simulink model "eBooster_48v_Gen2_r2009a"  (Simulink 7.6)
settings: Solver=FixedStepDiscrete  StartTime=0.0  StopTime=0.2  FixedStep=T_sim  RelTol=1e-3
InitFcn:
  | init_simulation
values from neighbouring files (symbols this model uses):
  C_Load = 0    [init_MIL.m]    (also in init_simulation.m)
  curr_adc_gain = 0.6247    [init_MIL.m]    (also in init_simulation.m)
  en_avr = 0    [init_MIL.m]    (also in init_simulation.m)
  FOC_CURR_GAIN_SCU10 = 640    [init_MIL.m]    (also in init_simulation.m)
  FOC_CURR_NULLIFICATION = 511    [init_MIL.m]    (also in init_simulation.m)
  I_max = 106    [init_MIL.m]    (also in init_simulation.m = 100; plot_current_limits.m = 160)
  Id_ref_min = -1*160*0.8    (= -128)    [init_MIL.m]    (also in init_simulation.m)
  J_motor = (3.2220 + 11.438)*1e-6    (= 1.466e-05)    [init_MIL.m]    (also in init_simulation.m)
  Kpi = 0.3    [init_MIL.m]    (also in init_simulation.m)
  Kpi_n = 0.0015    [init_MIL.m]    (also in init_simulation.m)
  load_motor_spd_ramp = (load_motor_target_spd - load_motor_start_spd)/spd_ramp_time    (= 62831.8530718)    [init_MIL.m]    (also in init_simulation.m)
  load_motor_start_spd = 40000*2*pi/60    (= 4188.79020479)    [init_MIL.m]    (also in init_simulation.m)
  load_motor_target_spd = 70000*2*pi/60    (= 7330.38285838)    [init_MIL.m]    (also in init_simulation.m)
  Ls = 17.05e-6/3    (= 5.68333333333e-06)    [init_MIL.m]    (also in init_simulation.m; plot_current_limits.m)
  N_avr = 1    [init_MIL.m]    (also in init_simulation.m)
  Nset_const = 50000    [init_MIL.m]    (also in init_simulation.m)
  ONEDIVSQRT3_SCU16 = 37837    [init_MIL.m]    (also in init_simulation.m)
  Pp = 1    [init_MIL.m]    (also in init_simulation.m; plot_current_limits.m)
  psi_p = 5.3e-3/sqrt(3)*0.95    [init_MIL.m]    (also in init_simulation.m)
  Rs = 10e-3*(1+0.0039*(120-20))/3    (= 0.00463333333333)    [init_MIL.m]    (also in init_simulation.m; plot_current_limits.m)
  Sel_Bench_Mode = 1    [init_MIL.m]    (also in init_simulation.m)
  Sel_Bench_Spd = 0    [init_MIL.m]    (also in init_simulation.m)
  Sel_id_ref = 2    [init_MIL.m]    (also in init_simulation.m)
  Sel_Load = 1    [init_MIL.m]    (also in init_simulation.m)
  sel_udq = 0    [init_simulation.m]
  Set_Speed_rpm = 50000    [init_MIL.m]    (also in init_simulation.m)
  T_ctrl = T_pwm    (= 3.57002606119e-05)    [init_MIL.m]    (also in init_simulation.m)
  T_LUT_T = [0.1864, 0.1969, 0.2092, 0.2230, 0.2381, 0.2541, 0.2709, 0.2880, 0.3054, 0.3226, 0.3395, 0.3557, 0.3710, 0.3851, 0.3978, 0.4088, 0.4178 ... (first row only)    [init_MIL.m]    (also in init_simulation.m)
  T_sim = T_pwm/100    (= 3.57002606119e-07)    [init_MIL.m]    (also in init_simulation.m)
  Tni = Ts    (= 0.00122661870504)    [init_MIL.m]    (also in init_simulation.m)
  Tni_n = Ts*1.5    (= 0.00183992805755)    [init_MIL.m]    (also in init_simulation.m)
  V_dc = 36    [init_MIL.m]    (also in init_simulation.m)
libraries: simulink x27
(part 1 of 2)
Description:
  | This model can be used to document and simulate the eBooster_Gen2_48V application including:
  | - Control algorithm
  | - Fix point scaling
  | - Interfaces (function arguments, global variables...)
  | 
  | File history:
settings Model: Creator=tree5_000  LastModifiedBy=meng
settings CodeAppCC: CustomSymbolStrType=$N$R$M_T

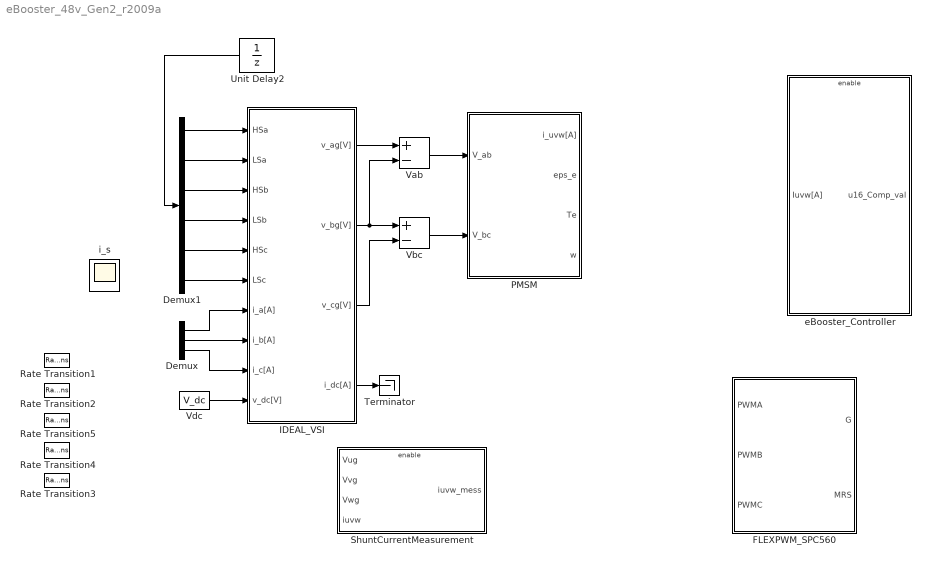
== system eBooster_48v_Gen2_r2009a ==
  Demux : Demux  Outputs=3
  Demux1 : Demux  Outputs=6
  FLEXPWM_SPC560 : Subsystem
  IDEAL_VSI : Subsystem
  PMSM : Subsystem  MinMaxOverflowLogging=ForceOff
  Rate Transition{1..5} (5 alike) : RateTransition  Integrity=off  Deterministic=off  OutPortSampleTime=T_ctrl
  ShuntCurrentMeasurement : Subsystem
  Terminator : Terminator
  Unit Delay2 : UnitDelay  SampleTime=-1
  Vab : Sum  Inputs=+-
  Vbc : Sum  Inputs=+-
  Vdc : Constant  Value=V_dc
  eBooster_Controller : Subsystem
  i_s : Scope
      settings: YMin=-500  YMax=500  SaveName=ScopeData2
  wires:
  IDEAL_VSI/1(v_ag[V]) -> Vab/1
  IDEAL_VSI/2(v_bg[V]) -> Vab/2, Vbc/1
  IDEAL_VSI/3(v_cg[V]) -> Vbc/2
  Vbc/1 -> PMSM/2(V_bc)
  Demux/1 -> IDEAL_VSI/7(i_a[A])
  Demux/2 -> IDEAL_VSI/8(i_b[A])
  Demux/3 -> IDEAL_VSI/9(i_c[A])
  Demux1/1 -> IDEAL_VSI/1(HSa)
  Demux1/2 -> IDEAL_VSI/2(LSa)
  Demux1/3 -> IDEAL_VSI/3(HSb)
  Demux1/4 -> IDEAL_VSI/4(LSb)
  Demux1/5 -> IDEAL_VSI/5(HSc)
  Demux1/6 -> IDEAL_VSI/6(LSc)
  IDEAL_VSI/4(i_dc[A]) -> Terminator/1
  Vab/1 -> PMSM/1(V_ab)
  Unit Delay2/1 -> Demux1/1
  Vdc/1 -> IDEAL_VSI/10(v_dc[V])

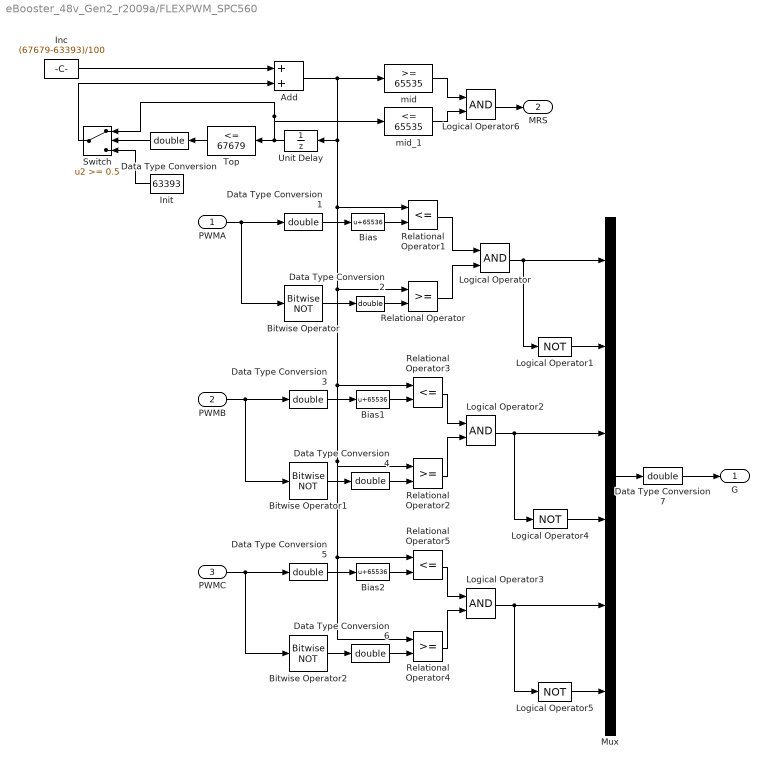
== system eBooster_48v_Gen2_r2009a/FLEXPWM_SPC560 ==
  PWMA : Inport
  PWMB : Inport  Port=2
  PWMC : Inport  Port=3
  Add : Sum
  Bias : Bias  Bias=65536
  Bias1 : Bias  Bias=65536
  Bias2 : Bias  Bias=65536
  Bitwise Operator : simulink/Logic and Bit Operations/Bitwise Operator  logicop=NOT  UseBitMask=off  BitMask=bin2dec('11011001')  BitMaskRealWorld=Stored Integer
  Bitwise Operator1 : simulink/Logic and Bit Operations/Bitwise Operator  logicop=NOT  UseBitMask=off  BitMask=bin2dec('11011001')  BitMaskRealWorld=Stored Integer
  Bitwise Operator2 : simulink/Logic and Bit Operations/Bitwise Operator  logicop=NOT  UseBitMask=off  BitMask=bin2dec('11011001')  BitMaskRealWorld=Stored Integer
  Data Type Conversion{,1..7} (8 alike) : DataTypeConversion  OutDataTypeStr=double
  Inc : Constant  Value=(67679-63393)/100
  Init : Constant  Value=63393
  Logical Operator{,2..3,6} (4 alike) : Logic  AllPortsSameDT=off  OutDataTypeStr=boolean
  Logical Operator1 : Logic  Operator=NOT  AllPortsSameDT=off  OutDataTypeStr=boolean
  Logical Operator4 : Logic  Operator=NOT  AllPortsSameDT=off  OutDataTypeStr=boolean
  Logical Operator5 : Logic  Operator=NOT  AllPortsSameDT=off  OutDataTypeStr=boolean
  Mux : Mux  Inputs=6
  Relational Operator : RelationalOperator  OutDataTypeStr=boolean
  Relational Operator1 : RelationalOperator  Operator=<=  OutDataTypeStr=boolean
  Relational Operator2 : RelationalOperator  OutDataTypeStr=boolean
  Relational Operator3 : RelationalOperator  Operator=<=  OutDataTypeStr=boolean
  Relational Operator4 : RelationalOperator  OutDataTypeStr=boolean
  Relational Operator5 : RelationalOperator  Operator=<=  OutDataTypeStr=boolean
  Switch : Switch  Threshold=0.5
  Top : simulink/Logic and Bit Operations/Compare To Constant  SystemSampleTime=-1  relop=<=  const=67679  LogicOutDataTypeMode=uint8  ZeroCross=off
  Unit Delay : UnitDelay  X0=63393  SampleTime=-1
  mid : simulink/Logic and Bit Operations/Compare To Constant  SystemSampleTime=-1  relop=>=  const=65535  LogicOutDataTypeMode=uint8  ZeroCross=off
  mid_1 : simulink/Logic and Bit Operations/Compare To Constant  SystemSampleTime=-1  relop=<=  const=65535  LogicOutDataTypeMode=uint8  ZeroCross=off
  G : Outport
  MRS : Outport  Port=2
  wires:
  Add/1 -> Unit Delay/1, Relational Operator1/1, Relational Operator/1, Relational Operator3/1, Relational Operator2/1, Relational Operator5/1, Relational Operator4/1, mid/1
  Inc/1 -> Add/1
  Unit Delay/1 -> Top/1, Switch/1, mid_1/1
  Top/1 -> Data Type Conversion/1
  Data Type Conversion/1 -> Switch/2
  Init/1 -> Switch/3
  Switch/1 -> Add/2
  Bitwise Operator/1 -> Data Type Conversion2/1
  PWMA/1 -> Data Type Conversion1/1, Bitwise Operator/1
  Bias/1 -> Relational Operator1/2
  Data Type Conversion1/1 -> Bias/1
  Data Type Conversion2/1 -> Relational Operator/2
  Relational Operator1/1 -> Logical Operator/1
  Relational Operator/1 -> Logical Operator/2
  Logical Operator/1 -> Logical Operator1/1, Mux/1
  Bitwise Operator1/1 -> Data Type Conversion4/1
  Bias1/1 -> Relational Operator3/2
  Data Type Conversion3/1 -> Bias1/1
  Data Type Conversion4/1 -> Relational Operator2/2
  Relational Operator3/1 -> Logical Operator2/1
  Relational Operator2/1 -> Logical Operator2/2
  Logical Operator2/1 -> Logical Operator4/1, Mux/3
  PWMB/1 -> Data Type Conversion3/1, Bitwise Operator1/1
  Bitwise Operator2/1 -> Data Type Conversion6/1
  Bias2/1 -> Relational Operator5/2
  Data Type Conversion5/1 -> Bias2/1
  Data Type Conversion6/1 -> Relational Operator4/2
  Relational Operator5/1 -> Logical Operator3/1
  Relational Operator4/1 -> Logical Operator3/2
  Logical Operator3/1 -> Mux/5, Logical Operator5/1
  PWMC/1 -> Bitwise Operator2/1, Data Type Conversion5/1
  Logical Operator1/1 -> Mux/2
  Logical Operator4/1 -> Mux/4
  Logical Operator5/1 -> Mux/6
  Mux/1 -> Data Type Conversion7/1
  Data Type Conversion7/1 -> G/1
  mid/1 -> Logical Operator6/1
  mid_1/1 -> Logical Operator6/2
  Logical Operator6/1 -> MRS/1

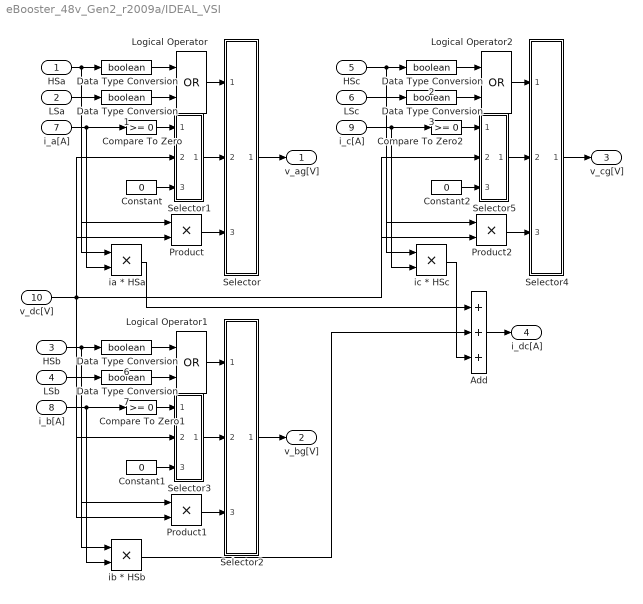
== system eBooster_48v_Gen2_r2009a/IDEAL_VSI ==
  HSa : Inport
  LSa : Inport  Port=2
  HSb : Inport  Port=3
  LSb : Inport  Port=4
  HSc : Inport  Port=5
  LSc : Inport  Port=6
  i_a[A] : Inport  Port=7
  i_b[A] : Inport  Port=8
  i_c[A] : Inport  Port=9
  v_dc[V] : Inport  Port=10
  Add : Sum  Inputs=+++
  Compare To Zero : simulink/Logic and Bit Operations/Compare To Zero  SystemSampleTime=-1  relop=>=  LogicOutDataTypeMode=uint8  ZeroCross=off
  Compare To Zero1 : simulink/Logic and Bit Operations/Compare To Zero  SystemSampleTime=-1  relop=>=  LogicOutDataTypeMode=uint8  ZeroCross=off
  Compare To Zero2 : simulink/Logic and Bit Operations/Compare To Zero  SystemSampleTime=-1  relop=>=  LogicOutDataTypeMode=uint8  ZeroCross=off
  Constant : Constant  Value=0
  Constant1 : Constant  Value=0
  Constant2 : Constant  Value=0
  Data Type Conversion{,1..3,6..7} (6 alike) : DataTypeConversion  OutDataTypeStr=boolean
  Logical Operator : Logic  Operator=OR  AllPortsSameDT=off  OutDataTypeStr=boolean
  Logical Operator1 : Logic  Operator=OR  AllPortsSameDT=off  OutDataTypeStr=boolean
  Logical Operator2 : Logic  Operator=OR  AllPortsSameDT=off  OutDataTypeStr=boolean
  Product : Product  RndMeth=Zero
  Product1 : Product  RndMeth=Zero
  Product2 : Product  RndMeth=Zero
  Selector : Subsystem
  Selector1 : Subsystem
  Selector2 : Subsystem
  Selector3 : Subsystem
  Selector4 : Subsystem
  Selector5 : Subsystem
  ia * HSa : Product  RndMeth=Zero
  ib * HSb : Product  RndMeth=Zero
  ic * HSc : Product  RndMeth=Zero
  v_ag[V] : Outport
  v_bg[V] : Outport  Port=2
  v_cg[V] : Outport  Port=3
  i_dc[A] : Outport  Port=4
  wires:
  HSa/1 -> Data Type Conversion/1, Product/1, ia * HSa/1
  LSa/1 -> Data Type Conversion1/1
  Data Type Conversion/1 -> Logical Operator/1
  Data Type Conversion1/1 -> Logical Operator/2
  Logical Operator/1 -> Selector/1(sel)
  i_a[A]/1 -> Compare To Zero/1, ia * HSa/2
  Compare To Zero/1 -> Selector1/1(sel)
  Constant/1 -> Selector1/3(d1)
  Selector1/1(" ") -> Selector/2(d0)
  v_dc[V]/1 -> Selector1/2(d0), Product/2, Selector3/2(d0), Product1/2, Selector5/2(d0), Product2/2
  Product/1 -> Selector/3(d1)
  Selector/1(" ") -> v_ag[V]/1
  HSb/1 -> Data Type Conversion6/1, Product1/1, ib * HSb/1
  LSb/1 -> Data Type Conversion7/1
  Data Type Conversion6/1 -> Logical Operator1/1
  Data Type Conversion7/1 -> Logical Operator1/2
  Logical Operator1/1 -> Selector2/1(sel)
  Compare To Zero1/1 -> Selector3/1(sel)
  Constant1/1 -> Selector3/3(d1)
  Selector3/1(" ") -> Selector2/2(d0)
  Product1/1 -> Selector2/3(d1)
  Selector2/1(" ") -> v_bg[V]/1
  i_b[A]/1 -> Compare To Zero1/1, ib * HSb/2
  HSc/1 -> Data Type Conversion2/1, Product2/1, ic * HSc/1
  LSc/1 -> Data Type Conversion3/1
  Data Type Conversion2/1 -> Logical Operator2/1
  Data Type Conversion3/1 -> Logical Operator2/2
  Logical Operator2/1 -> Selector4/1(sel)
  Compare To Zero2/1 -> Selector5/1(sel)
  Constant2/1 -> Selector5/3(d1)
  Selector5/1(" ") -> Selector4/2(d0)
  Product2/1 -> Selector4/3(d1)
  Selector4/1(" ") -> v_cg[V]/1
  i_c[A]/1 -> Compare To Zero2/1, ic * HSc/2
  ic * HSc/1 -> Add/3
  ia * HSa/1 -> Add/1
  ib * HSb/1 -> Add/2
  Add/1 -> i_dc[A]/1

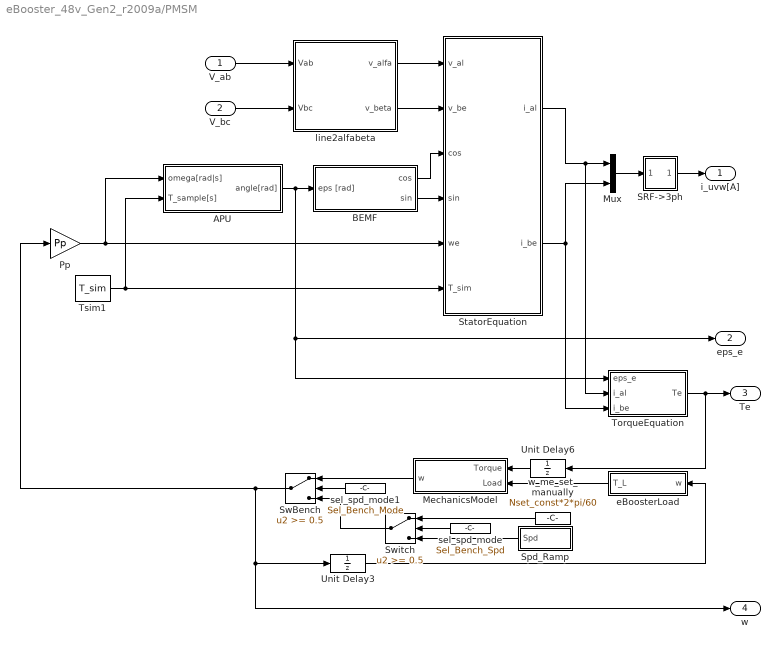
== system eBooster_48v_Gen2_r2009a/PMSM ==
  V_ab : Inport
  V_bc : Inport  Port=2
  APU : Subsystem
  BEMF : Subsystem
  MechanicsModel : Subsystem
  Mux : Mux  Inputs=2
  Pp : Gain  Gain=Pp
  SRF->3ph : Subsystem
  Spd_Ramp : Subsystem
  StatorEquation : Subsystem  MinMaxOverflowLogging=MinMaxAndOverflow
  SwBench : Switch  Threshold=0.5
  Switch : Switch  Threshold=0.5
  TorqueEquation : Subsystem
  Tsim1 : Constant  Value=T_sim
  Unit Delay3 : UnitDelay  SampleTime=-1
  Unit Delay6 : UnitDelay  SampleTime=-1
  eBoosterLoad : Subsystem
  line2alfabeta : Subsystem
  sel_spd_mode : Constant  Value=Sel_Bench_Spd
  sel_spd_mode1 : Constant  Value=Sel_Bench_Mode
  w_me_set_manually : Constant  Value=Nset_const*2*pi/60
  i_uvw[A] : Outport
  eps_e : Outport  Port=2
  Te : Outport  Port=3
  w : Outport  Port=4
  wires:
  APU/1(angle[rad]) -> BEMF/1(eps [rad]), TorqueEquation/1(eps_e), eps_e/1
  line2alfabeta/1(v_alfa) -> StatorEquation/1(v_al)
  line2alfabeta/2(v_beta) -> StatorEquation/2(v_be)
  BEMF/1(cos) -> StatorEquation/3(cos)
  BEMF/2(sin) -> StatorEquation/4(sin)
  Pp/1 -> StatorEquation/5(we), APU/1(omega[rad|s])
  V_ab/1 -> line2alfabeta/1(Vab)
  V_bc/1 -> line2alfabeta/2(Vbc)
  Tsim1/1 -> StatorEquation/6(T_sim), APU/2(T_sample[s])
  TorqueEquation/1(Te) -> Te/1, Unit Delay6/1
  SRF->3ph/1(abc) -> i_uvw[A]/1
  Mux/1 -> SRF->3ph/1(alpha beta)
  StatorEquation/1(i_al) -> Mux/1, TorqueEquation/2(i_al)
  StatorEquation/2(i_be) -> Mux/2, TorqueEquation/3(i_be)
  Switch/1 -> SwBench/3
  w_me_set_manually/1 -> Switch/1
  Spd_Ramp/1(Spd) -> Switch/3
  sel_spd_mode/1 -> Switch/2
  sel_spd_mode1/1 -> SwBench/2
  MechanicsModel/1(w) -> SwBench/1
  SwBench/1 -> Pp/1, Unit Delay3/1, w/1
  eBoosterLoad/1(T_L) -> MechanicsModel/2(Load)
  Unit Delay3/1 -> eBoosterLoad/1(w)
  Unit Delay6/1 -> MechanicsModel/1(Torque)

== system eBooster_48v_Gen2_r2009a/ShuntCurrentMeasurement ==
  Vug : Inport
  Vvg : Inport  Port=2
  Vwg : Inport  Port=3
  iuvw : Inport  Port=4
  Enable : EnablePort
  Demux : Demux  Outputs=3
  Gain : Gain  Gain=-1
  Mux : Mux  Inputs=3
  NoMeasurement : Constant  Value=0
  Switch : Switch  Threshold=0.5
  Switch1 : Switch  Threshold=0.5
  Switch2 : Switch  Threshold=0.5
  isZero : simulink/Logic and Bit Operations/Compare To Zero  SystemSampleTime=-1  relop=~=  LogicOutDataTypeMode=uint8  ZeroCross=off
  isZero1 : simulink/Logic and Bit Operations/Compare To Zero  SystemSampleTime=-1  relop=~=  LogicOutDataTypeMode=uint8  ZeroCross=off
  isZero2 : simulink/Logic and Bit Operations/Compare To Zero  SystemSampleTime=-1  relop=~=  LogicOutDataTypeMode=uint8  ZeroCross=off
  iuvw_mess : Outport
  wires:
  iuvw/1 -> Gain/1
  Gain/1 -> Demux/1
  NoMeasurement/1 -> Switch/1, Switch1/1, Switch2/1
  Demux/1 -> Switch/3
  Demux/2 -> Switch1/3
  Demux/3 -> Switch2/3
  Vug/1 -> isZero/1
  Vvg/1 -> isZero1/1
  Vwg/1 -> isZero2/1
  isZero/1 -> Switch/2
  isZero1/1 -> Switch1/2
  isZero2/1 -> Switch2/2
  Switch/1 -> Mux/1
  Switch1/1 -> Mux/2
  Switch2/1 -> Mux/3
  Mux/1 -> iuvw_mess/1

== system eBooster_48v_Gen2_r2009a/eBooster_Controller ==
  note: N_{ref} as rpm in uint32
  Iuvw[A] : Inport
  Enable : EnablePort
  FOC_Calc : Subsystem
  MeasurementAndScaling : Subsystem
  SpeedSet : Constant  Value=Set_Speed_rpm  OutDataTypeStr=uint32
  init_se_Sector : UnitDelay  X0=1  SampleTime=-1
  u16_Comp_val : Outport
  wires:
  ? -> u16_Comp_val/1
  init_se_Sector/1 -> MeasurementAndScaling/4(se_Sector)
  MeasurementAndScaling/1(s_s16_I_alpha) -> FOC_Calc/1(s_s16_I_alpha)
  MeasurementAndScaling/2(s_s16_I_beta) -> FOC_Calc/2(s_s16_I_beta)
  MeasurementAndScaling/3(u16_Umeas_V_dig) -> FOC_Calc/3(u16_Umeas_V_dig)
  MeasurementAndScaling/4(g_u32_V_48) -> FOC_Calc/4(g_u32_V_48)
  SpeedSet/1 -> FOC_Calc/5(u32_DesiredCANSpeed)
  Iuvw[A]/1 -> MeasurementAndScaling/1(Iuvw[A])

== system eBooster_48v_Gen2_r2009a/IDEAL_VSI/Selector ==
  sel : Inport
  d0 : Inport  Port=2
  d1 : Inport  Port=3
  If : If  IfExpression=u1 == 0
  If Action Subsystem : Subsystem  TreatAsAtomicUnit=on
  If Action Subsystem1 : Subsystem  TreatAsAtomicUnit=on
  Merge : Merge
  " " : Outport
  wires:
  sel/1 -> If/1
  If/1 -> If Action Subsystem/Action
  d0/1 -> If Action Subsystem/1(In1)
  d1/1 -> If Action Subsystem1/1(In1)
  If/2 -> If Action Subsystem1/Action
  If Action Subsystem/1(Out1) -> Merge/1
  If Action Subsystem1/1(Out1) -> Merge/2
  Merge/1 -> " "/1

== system eBooster_48v_Gen2_r2009a/IDEAL_VSI/Selector1 ==
  sel : Inport
  d0 : Inport  Port=2
  d1 : Inport  Port=3
  If : If  IfExpression=u1 == 0
  If Action Subsystem : Subsystem  TreatAsAtomicUnit=on
  If Action Subsystem1 : Subsystem  TreatAsAtomicUnit=on
  Merge : Merge
  " " : Outport
  wires:
  Merge/1 -> " "/1
  If Action Subsystem1/1(Out1) -> Merge/2
  If Action Subsystem/1(Out1) -> Merge/1
  If/2 -> If Action Subsystem1/Action
  d1/1 -> If Action Subsystem1/1(In1)
  d0/1 -> If Action Subsystem/1(In1)
  If/1 -> If Action Subsystem/Action
  sel/1 -> If/1

== system eBooster_48v_Gen2_r2009a/IDEAL_VSI/Selector2 ==
  sel : Inport
  d0 : Inport  Port=2
  d1 : Inport  Port=3
  If : If  IfExpression=u1 == 0
  If Action Subsystem : Subsystem  TreatAsAtomicUnit=on
  If Action Subsystem1 : Subsystem  TreatAsAtomicUnit=on
  Merge : Merge
  " " : Outport
  wires:
  sel/1 -> If/1
  If/1 -> If Action Subsystem/Action
  d0/1 -> If Action Subsystem/1(In1)
  d1/1 -> If Action Subsystem1/1(In1)
  If/2 -> If Action Subsystem1/Action
  If Action Subsystem/1(Out1) -> Merge/1
  If Action Subsystem1/1(Out1) -> Merge/2
  Merge/1 -> " "/1

== system eBooster_48v_Gen2_r2009a/IDEAL_VSI/Selector3 ==
  sel : Inport
  d0 : Inport  Port=2
  d1 : Inport  Port=3
  If : If  IfExpression=u1 == 0
  If Action Subsystem : Subsystem  TreatAsAtomicUnit=on
  If Action Subsystem1 : Subsystem  TreatAsAtomicUnit=on
  Merge : Merge
  " " : Outport
  wires:
  Merge/1 -> " "/1
  If Action Subsystem1/1(Out1) -> Merge/2
  If Action Subsystem/1(Out1) -> Merge/1
  If/2 -> If Action Subsystem1/Action
  d1/1 -> If Action Subsystem1/1(In1)
  d0/1 -> If Action Subsystem/1(In1)
  If/1 -> If Action Subsystem/Action
  sel/1 -> If/1

== system eBooster_48v_Gen2_r2009a/IDEAL_VSI/Selector4 ==
  sel : Inport
  d0 : Inport  Port=2
  d1 : Inport  Port=3
  If : If  IfExpression=u1 == 0
  If Action Subsystem : Subsystem  TreatAsAtomicUnit=on
  If Action Subsystem1 : Subsystem  TreatAsAtomicUnit=on
  Merge : Merge
  " " : Outport
  wires:
  sel/1 -> If/1
  If/1 -> If Action Subsystem/Action
  d0/1 -> If Action Subsystem/1(In1)
  d1/1 -> If Action Subsystem1/1(In1)
  If/2 -> If Action Subsystem1/Action
  If Action Subsystem/1(Out1) -> Merge/1
  If Action Subsystem1/1(Out1) -> Merge/2
  Merge/1 -> " "/1

== system eBooster_48v_Gen2_r2009a/IDEAL_VSI/Selector5 ==
  sel : Inport
  d0 : Inport  Port=2
  d1 : Inport  Port=3
  If : If  IfExpression=u1 == 0
  If Action Subsystem : Subsystem  TreatAsAtomicUnit=on
  If Action Subsystem1 : Subsystem  TreatAsAtomicUnit=on
  Merge : Merge
  " " : Outport
  wires:
  Merge/1 -> " "/1
  If Action Subsystem1/1(Out1) -> Merge/2
  If Action Subsystem/1(Out1) -> Merge/1
  If/2 -> If Action Subsystem1/Action
  d1/1 -> If Action Subsystem1/1(In1)
  d0/1 -> If Action Subsystem/1(In1)
  If/1 -> If Action Subsystem/Action
  sel/1 -> If/1

== system eBooster_48v_Gen2_r2009a/PMSM/APU ==
  note: Unit delay is viewed equivalent to register in XSG
  omega[rad|s] : Inport
  T_sample[s] : Inport  Port=2
  Add : Sum  OutDataTypeStr=Inherit: Same as first input
  Compare To Constant : simulink/Logic and Bit Operations/Compare To Constant  SystemSampleTime=-1  relop=>=  const=2*pi  LogicOutDataTypeMode=uint8  ZeroCross=off
  Constant : Constant  Value=0
  Data Type Conversion : DataTypeConversion  OutDataTypeStr=double
  Multiport Switch : MultiPortSwitch  DataPortOrder=Zero-based contiguous  Inputs=2  zeroidx=on
  Product : Product  RndMeth=Zero
  Unit Delay : UnitDelay  SampleTime=-1
  angle[rad] : Outport
  wires:
  Constant/1 -> Multiport Switch/3
  Multiport Switch/1 -> angle[rad]/1, Unit Delay/1
  Data Type Conversion/1 -> Multiport Switch/1
  Compare To Constant/1 -> Data Type Conversion/1
  Add/1 -> Multiport Switch/2, Compare To Constant/1
  Product/1 -> Add/1
  Unit Delay/1 -> Add/2
  omega[rad|s]/1 -> Product/1
  T_sample[s]/1 -> Product/2

== system eBooster_48v_Gen2_r2009a/PMSM/BEMF ==
  eps [rad] : Inport
  Trigonometric Function : Trigonometry
  Trigonometric Function1 : Trigonometry  Operator=cos
  cos : Outport
  sin : Outport  Port=2
  wires:
  eps [rad]/1 -> Trigonometric Function1/1, Trigonometric Function/1
  Trigonometric Function/1 -> sin/1
  Trigonometric Function1/1 -> cos/1

== system eBooster_48v_Gen2_r2009a/PMSM/MechanicsModel ==
  Torque : Inport
  Load : Inport  Port=2
  Add : Sum
  Subtract : Sum  Inputs=+-
  Unit Delay : UnitDelay  SampleTime=-1
  dw_dt*dT : Gain  Gain=1/J_motor*T_sim
  w : Outport
  wires:
  Add/1 -> Unit Delay/1, w/1
  Unit Delay/1 -> Add/2
  dw_dt*dT/1 -> Add/1
  Subtract/1 -> dw_dt*dT/1
  Torque/1 -> Subtract/1
  Load/1 -> Subtract/2

== system eBooster_48v_Gen2_r2009a/PMSM/SRF->3ph ==
  alpha beta : Inport  PortDimensions=2
  Mux : Mux  Inputs=3
  a : Fcn  Expr=u[1]
  b : Fcn  Expr=(-u[1]+sqrt(3)*u[2])/2
  c : Fcn  Expr=(-u[1]-sqrt(3)*u[2])/2
  abc : Outport
  wires:
  alpha beta/1 -> c/1, a/1, b/1
  Mux/1 -> abc/1
  c/1 -> Mux/3
  b/1 -> Mux/2
  a/1 -> Mux/1

== system eBooster_48v_Gen2_r2009a/PMSM/Spd_Ramp ==
  Ramp : simulink/Sources/Ramp  SystemSampleTime=-1  slope=load_motor_spd_ramp  start=0  X0=load_motor_start_spd
  Rate Transition : RateTransition  OutPortSampleTime=T_sim
  Saturation : Saturate  UpperLimit=load_motor_target_spd  LowerLimit=0
  Spd : Outport
  wires:
  Rate Transition/1 -> Spd/1
  Saturation/1 -> Rate Transition/1
  Ramp/1 -> Saturation/1

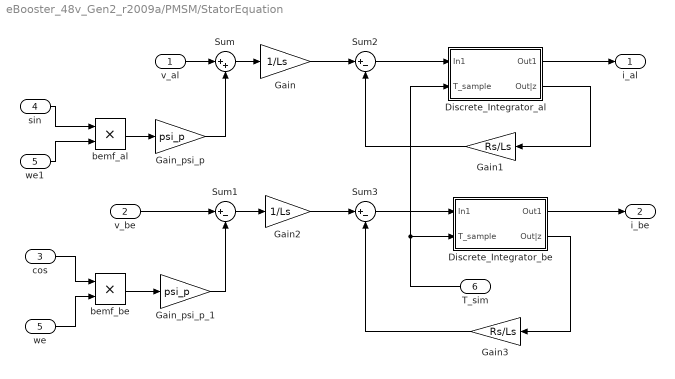
== system eBooster_48v_Gen2_r2009a/PMSM/StatorEquation ==
  v_al : Inport
  v_be : Inport  Port=2
  cos : Inport  Port=3
  sin : Inport  Port=4
  we : Inport  Port=5
  T_sim : Inport  Port=6
  Discrete_Integrator_al : Subsystem
  Discrete_Integrator_be : Subsystem
  Gain : Gain  Gain=1/Ls  OutDataTypeStr=double
  Gain1 : Gain  Gain=Rs/Ls  OutDataTypeStr=double
  Gain2 : Gain  Gain=1/Ls  OutDataTypeStr=double
  Gain3 : Gain  Gain=Rs/Ls  OutDataTypeStr=double
  Gain_psi_p : Gain  Gain=psi_p  OutDataTypeStr=double
  Gain_psi_p_1 : Gain  Gain=psi_p  OutDataTypeStr=double
  Sum : Sum  Inputs=|++
  Sum1 : Sum  Inputs=|+-
  Sum2 : Sum  Inputs=|+-
  Sum3 : Sum  Inputs=|+-
  bemf_al : Product  OutDataTypeStr=double  RndMeth=Zero
  bemf_be : Product  OutDataTypeStr=double  RndMeth=Zero
  we1 : InportShadow  Port=5
  i_al : Outport
  i_be : Outport  Port=2
  wires:
  Sum/1 -> Gain/1
  Gain/1 -> Sum2/1
  Sum2/1 -> Discrete_Integrator_al/1(In1)
  Sum1/1 -> Gain2/1
  Gain2/1 -> Sum3/1
  Sum3/1 -> Discrete_Integrator_be/1(In1)
  T_sim/1 -> Discrete_Integrator_al/2(T_sample), Discrete_Integrator_be/2(T_sample)
  Discrete_Integrator_al/1(Out1) -> i_al/1
  Discrete_Integrator_be/1(Out1) -> i_be/1
  Discrete_Integrator_al/2(Out|z) -> Gain1/1
  Gain1/1 -> Sum2/2
  Discrete_Integrator_be/2(Out|z) -> Gain3/1
  Gain3/1 -> Sum3/2
  cos/1 -> bemf_be/1
  we/1 -> bemf_be/2
  bemf_be/1 -> Gain_psi_p_1/1
  sin/1 -> bemf_al/1
  we1/1 -> bemf_al/2
  bemf_al/1 -> Gain_psi_p/1
  Gain_psi_p/1 -> Sum/2
  Gain_psi_p_1/1 -> Sum1/2
  v_al/1 -> Sum/1
  v_be/1 -> Sum1/1

== system eBooster_48v_Gen2_r2009a/PMSM/TorqueEquation ==
  eps_e : Inport
  i_al : Inport  Port=2
  i_be : Inport  Port=3
  Add : Sum  Inputs=+-
  Gain : Gain  Gain=psi_p
  Gain1 : Gain  Gain=psi_p
  Gain2 : Gain  Gain=1.5*Pp
  Product : Product  RndMeth=Zero
  Product1 : Product  RndMeth=Zero
  psi_al : Trigonometry  Operator=cos
  psi_al1 : Trigonometry
  Te : Outport
  wires:
  psi_al/1 -> Gain/1
  eps_e/1 -> psi_al/1, psi_al1/1
  Gain/1 -> Product/1
  psi_al1/1 -> Gain1/1
  i_be/1 -> Product/2
  Gain1/1 -> Product1/1
  i_al/1 -> Product1/2
  Product/1 -> Add/1
  Product1/1 -> Add/2
  Add/1 -> Gain2/1
  Gain2/1 -> Te/1

== system eBooster_48v_Gen2_r2009a/PMSM/eBoosterLoad ==
  w : Inport
  C_Load : Constant  Value=C_Load
  LUT_Load_eBooster : Lookup2D  RowIndex=T_LUT_row_ind  ColumnIndex=T_LUT_col_ind  Table=T_LUT_T
  Switch : Switch  Threshold=0.5
  massflow : Constant  Value=0.035
  sel : Constant  Value=Sel_Load
  T_L : Outport
  wires:
  w/1 -> LUT_Load_eBooster/1
  massflow/1 -> LUT_Load_eBooster/2
  Switch/1 -> T_L/1
  LUT_Load_eBooster/1 -> Switch/1
  sel/1 -> Switch/2
  C_Load/1 -> Switch/3

== system eBooster_48v_Gen2_r2009a/PMSM/line2alfabeta ==
  Vab : Inport
  Vbc : Inport  Port=2
  Add : Sum
  Gain : Gain  Gain=2
  Gain1 : Gain  Gain=1/3
  Gain2 : Gain  Gain=1/sqrt(3)
  v_alfa : Outport
  v_beta : Outport  Port=2
  wires:
  Gain2/1 -> v_beta/1
  Gain1/1 -> v_alfa/1
  Add/1 -> Gain1/1
  Vbc/1 -> Gain2/1, Add/2
  Gain/1 -> Add/1
  Vab/1 -> Gain/1

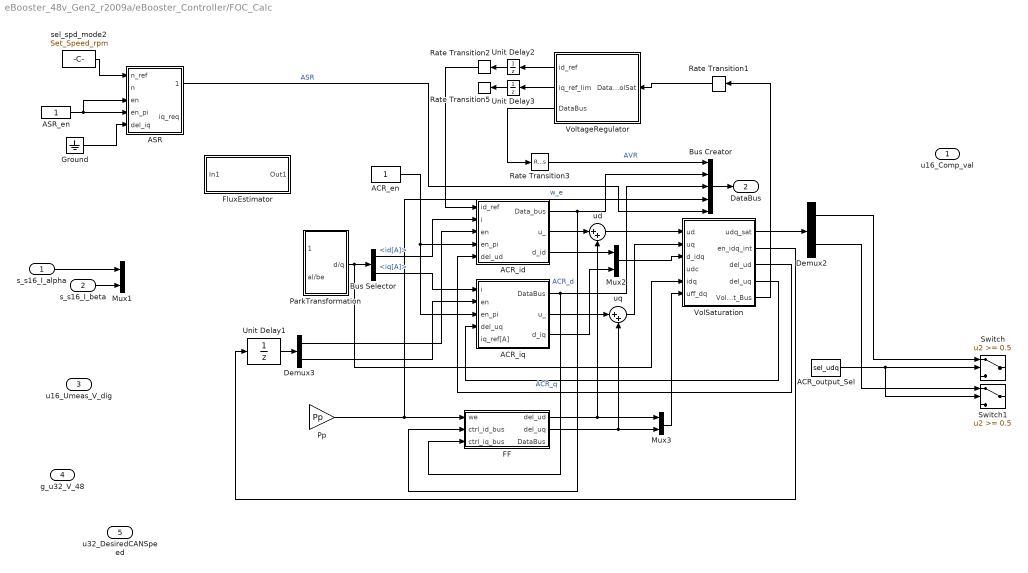
== system eBooster_48v_Gen2_r2009a/eBooster_Controller/FOC_Calc ==
  s_s16_I_alpha : Inport
  s_s16_I_beta : Inport  Port=2
  u16_Umeas_V_dig : Inport  Port=3
  g_u32_V_48 : Inport  Port=4
  u32_DesiredCANSpeed : Inport  Port=5
  ACR_en : Constant  SampleTime=T_ctrl
  ACR_id : Subsystem
  ACR_iq : Subsystem
  ACR_output_Sel : Constant  Value=sel_udq  SampleTime=T_ctrl
  ASR : Subsystem
  ASR_en : Constant  SampleTime=T_ctrl
  Bus Creator : BusCreator  Inputs=5
  Bus Selector : BusSelector  OutputSignals=id[A],iq[A]
  Demux2 : Demux  Outputs=2
  Demux3 : Demux  Outputs=2
  FF : Subsystem
  FluxEstimator : Subsystem
  Ground : Ground
  Mux1 : Mux  Inputs=2
  Mux2 : Mux  Inputs=2
  Mux3 : Mux  Inputs=2
  ParkTransformation : Subsystem
  Pp : Gain  Gain=Pp
  Rate Transition1 : RateTransition  Integrity=off  Deterministic=off  OutPortSampleTime=T_ctrl*N_avr
  Rate Transition2 : RateTransition  Integrity=off  Deterministic=off  OutPortSampleTime=T_ctrl
  Rate Transition3 : RateTransition  Integrity=off  Deterministic=off  OutPortSampleTime=T_ctrl
  Rate Transition5 : RateTransition  Integrity=off  Deterministic=off  OutPortSampleTime=T_ctrl
  Switch : Switch  Threshold=0.5
  Switch1 : Switch  Threshold=0.5
  Unit Delay1 : UnitDelay  SampleTime=T_ctrl
  Unit Delay2 : UnitDelay  SampleTime=-1
  Unit Delay3 : UnitDelay  SampleTime=-1
  VolSaturation : Subsystem
  VoltageRegulator : Subsystem  TreatAsAtomicUnit=on
  sel_spd_mode2 : Constant  Value=Set_Speed_rpm
  ud : Sum  Inputs=|++
  uq : Sum  Inputs=|++
  u16_Comp_val : Outport
  DataBus : Outport  Port=2
  wires:
  s_s16_I_alpha/1 -> Mux1/1
  s_s16_I_beta/1 -> Mux1/2
  Bus Selector/1 -> ACR_id/2(i)  "<id[A]>"
  Bus Selector/2 -> ACR_iq/1(i)  "<iq[A]>"
  ACR_id/2(u_) -> ud/1
  ACR_iq/2(u_) -> uq/1
  ud/1 -> VolSaturation/1(ud)
  uq/1 -> VolSaturation/2(uq)
  VolSaturation/1(udq_sat) -> Demux2/1
  Demux3/1 -> ACR_id/3(en)
  Demux3/2 -> ACR_iq/2(en)
  Unit Delay1/1 -> Demux3/1
  ACR_id/3(d_id) -> Mux2/1
  ACR_iq/3(d_iq) -> Mux2/2
  Mux2/1 -> VolSaturation/3(d_idq)
  Mux3/1 -> VolSaturation/6(uff_dq)
  FF/1(del_ud) -> Mux3/1, ud/2
  FF/2(del_uq) -> Mux3/2, uq/2
  VolSaturation/3(del_ud) -> ACR_id/5(del_ud)
  VolSaturation/4(del_uq) -> ACR_iq/4(del_uq)
  VolSaturation/2(en_idq_int) -> Unit Delay1/1
  ACR_en/1 -> ACR_id/4(en_pi), ACR_iq/3(en_pi)
  VolSaturation/5(VolSat_Bus) -> Rate Transition1/1
  Rate Transition1/1 -> VoltageRegulator/1(DataBusVolSat)
  VoltageRegulator/1(id_ref) -> Unit Delay2/1
  Unit Delay2/1 -> Rate Transition2/1
  Rate Transition2/1 -> ACR_id/1(id_ref)
  VoltageRegulator/3(DataBus) -> Rate Transition3/1
  Rate Transition3/1 -> Bus Creator/1  "AVR"
  ACR_id/1(Data_bus) -> FF/2(ctrl_id_bus), Bus Creator/2  "ACR_d"
  ACR_iq/1(DataBus) -> FF/3(ctrl_iq_bus), Bus Creator/3  "ACR_q"
  Bus Creator/1 -> DataBus/1
  VoltageRegulator/2(iq_ref_lim) -> Unit Delay3/1
  Unit Delay3/1 -> Rate Transition5/1
  Demux2/1 -> Switch/1
  Demux2/2 -> Switch1/1
  ACR_output_Sel/1 -> Switch/2, Switch1/2
  ParkTransformation/1(d/q) -> Bus Selector/1, VolSaturation/5(idq)
  ASR_en/1 -> ASR/4(en_pi), ASR/3(en)
  sel_spd_mode2/1 -> ASR/1(n_ref)
  Ground/1 -> ASR/5(del_iq)
  Pp/1 -> FF/1(we), Bus Creator/4  "w_e"
  ASR/1(Data_bus) -> Bus Creator/5  "ASR"

== system eBooster_48v_Gen2_r2009a/eBooster_Controller/MeasurementAndScaling ==
  Iuvw[A] : Inport
  Uuvw[V] : Inport  Port=2
  KL40[V] : Inport  Port=3
  se_Sector : Inport  Port=4
  Iuvw_Meas1 : Subsystem
  _0_ADC_EVALUATION _1_CLARKE_TRANSFORMATION1 : Subsystem
  s_s16_I_alpha : Outport
  s_s16_I_beta : Outport  Port=2
  u16_Umeas_V_dig : Outport  Port=3
  g_u32_V_48 : Outport  Port=4
  wires:
  KL40[V]/1 -> g_u32_V_48/1
  Iuvw[A]/1 -> Iuvw_Meas1/1(Iuvw[A])
  Iuvw_Meas1/1(S16_Iuvw_ADC) -> _0_ADC_EVALUATION _1_CLARKE_TRANSFORMATION1/2(i_uvw_adc)
  se_Sector/1 -> _0_ADC_EVALUATION _1_CLARKE_TRANSFORMATION1/1(se_Sector)
  _0_ADC_EVALUATION _1_CLARKE_TRANSFORMATION1/1(s_s16_I_alpha) -> s_s16_I_alpha/1
  _0_ADC_EVALUATION _1_CLARKE_TRANSFORMATION1/2(s_s16_I_beta) -> s_s16_I_beta/1

== system eBooster_48v_Gen2_r2009a/IDEAL_VSI/Selector/If Action Subsystem ==
  In1 : Inport
  Action Port : ActionPort  PropagateVarSize=During execution  ActionType=then
  Out1 : Outport
  wires:
  In1/1 -> Out1/1

== system eBooster_48v_Gen2_r2009a/IDEAL_VSI/Selector/If Action Subsystem1 ==
  In1 : Inport
  Action Port : ActionPort  PropagateVarSize=During execution  ActionType=else
  Out1 : Outport
  wires:
  In1/1 -> Out1/1

== system eBooster_48v_Gen2_r2009a/IDEAL_VSI/Selector1/If Action Subsystem ==
  In1 : Inport
  Action Port : ActionPort  PropagateVarSize=During execution  ActionType=then
  Out1 : Outport
  wires:
  In1/1 -> Out1/1

== system eBooster_48v_Gen2_r2009a/IDEAL_VSI/Selector1/If Action Subsystem1 ==
  In1 : Inport
  Action Port : ActionPort  PropagateVarSize=During execution  ActionType=else
  Out1 : Outport
  wires:
  In1/1 -> Out1/1

== system eBooster_48v_Gen2_r2009a/IDEAL_VSI/Selector2/If Action Subsystem ==
  In1 : Inport
  Action Port : ActionPort  PropagateVarSize=During execution  ActionType=then
  Out1 : Outport
  wires:
  In1/1 -> Out1/1

== system eBooster_48v_Gen2_r2009a/IDEAL_VSI/Selector2/If Action Subsystem1 ==
  In1 : Inport
  Action Port : ActionPort  PropagateVarSize=During execution  ActionType=else
  Out1 : Outport
  wires:
  In1/1 -> Out1/1

== system eBooster_48v_Gen2_r2009a/IDEAL_VSI/Selector3/If Action Subsystem ==
  In1 : Inport
  Action Port : ActionPort  PropagateVarSize=During execution  ActionType=then
  Out1 : Outport
  wires:
  In1/1 -> Out1/1

== system eBooster_48v_Gen2_r2009a/IDEAL_VSI/Selector3/If Action Subsystem1 ==
  In1 : Inport
  Action Port : ActionPort  PropagateVarSize=During execution  ActionType=else
  Out1 : Outport
  wires:
  In1/1 -> Out1/1

== system eBooster_48v_Gen2_r2009a/IDEAL_VSI/Selector4/If Action Subsystem ==
  In1 : Inport
  Action Port : ActionPort  PropagateVarSize=During execution  ActionType=then
  Out1 : Outport
  wires:
  In1/1 -> Out1/1

== system eBooster_48v_Gen2_r2009a/IDEAL_VSI/Selector4/If Action Subsystem1 ==
  In1 : Inport
  Action Port : ActionPort  PropagateVarSize=During execution  ActionType=else
  Out1 : Outport
  wires:
  In1/1 -> Out1/1

== system eBooster_48v_Gen2_r2009a/IDEAL_VSI/Selector5/If Action Subsystem ==
  In1 : Inport
  Action Port : ActionPort  PropagateVarSize=During execution  ActionType=then
  Out1 : Outport
  wires:
  In1/1 -> Out1/1

== system eBooster_48v_Gen2_r2009a/IDEAL_VSI/Selector5/If Action Subsystem1 ==
  In1 : Inport
  Action Port : ActionPort  PropagateVarSize=During execution  ActionType=else
  Out1 : Outport
  wires:
  In1/1 -> Out1/1

== system eBooster_48v_Gen2_r2009a/PMSM/StatorEquation/Discrete_Integrator_al ==
  note: Unit delay is viewed equivalent to register in XSG
  In1 : Inport
  T_sample : Inport  Port=2
  Add : Sum  OutDataTypeStr=double
  Data Type Conversion : DataTypeConversion  OutDataTypeStr=double
  Data Type Conversion1 : DataTypeConversion  OutDataTypeStr=double
  Product : Product  OutDataTypeStr=double  RndMeth=Zero
  Unit Delay : UnitDelay  SampleTime=-1
  Out1 : Outport
  Out|z : Outport  Port=2
  wires:
  T_sample/1 -> Product/2
  Product/1 -> Add/1
  Unit Delay/1 -> Add/2, Data Type Conversion1/1
  Add/1 -> Unit Delay/1, Data Type Conversion/1
  In1/1 -> Product/1
  Data Type Conversion/1 -> Out1/1
  Data Type Conversion1/1 -> Out|z/1

== system eBooster_48v_Gen2_r2009a/PMSM/StatorEquation/Discrete_Integrator_be ==
  note: Unit delay is viewed equivalent to register in XSG
  In1 : Inport
  T_sample : Inport  Port=2
  Add : Sum  OutDataTypeStr=double
  Data Type Conversion : DataTypeConversion  OutDataTypeStr=double
  Data Type Conversion1 : DataTypeConversion  OutDataTypeStr=double
  Product : Product  OutDataTypeStr=double  RndMeth=Zero
  Unit Delay : UnitDelay  SampleTime=-1
  Out1 : Outport
  Out|z : Outport  Port=2
  wires:
  Data Type Conversion1/1 -> Out|z/1
  Data Type Conversion/1 -> Out1/1
  In1/1 -> Product/1
  Add/1 -> Data Type Conversion/1, Unit Delay/1
  Unit Delay/1 -> Data Type Conversion1/1, Add/2
  Product/1 -> Add/1
  T_sample/1 -> Product/2

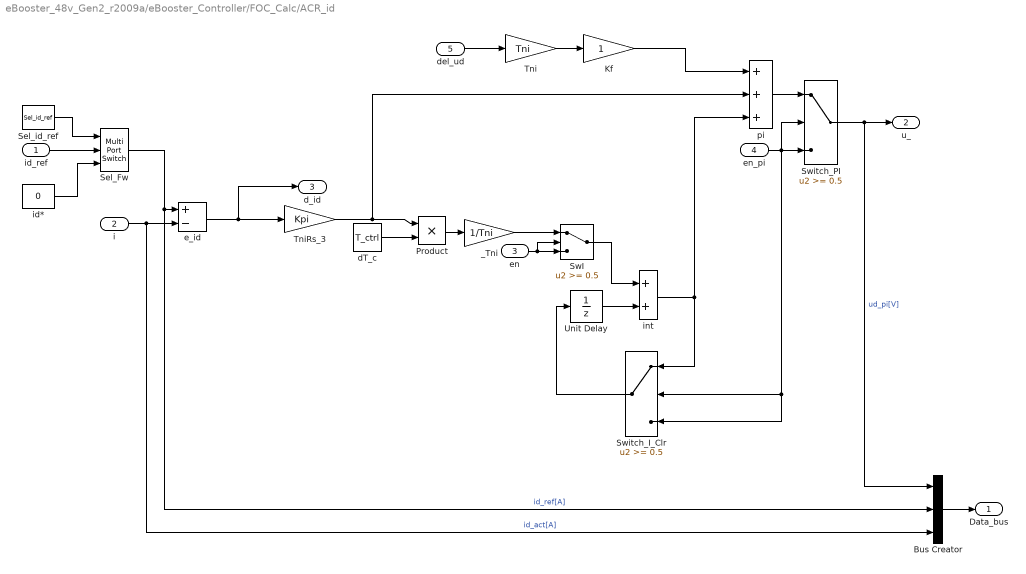
== system eBooster_48v_Gen2_r2009a/eBooster_Controller/FOC_Calc/ACR_id ==
  id_ref : Inport
  i : Inport  Port=2
  en : Inport  Port=3
  en_pi : Inport  Port=4
  del_ud : Inport  Port=5
  Bus Creator : BusCreator  Inputs=3
  Kf : Gain
  Product : Product  RndMeth=Zero
  Sel_Fw : MultiPortSwitch  Inputs=2  zeroidx=off
  Sel_id_ref : Constant  Value=Sel_id_ref  SampleTime=T_ctrl
  SwI : Switch  Threshold=0.5
  Switch_I_Clr : Switch  Threshold=0.5
  Switch_PI : Switch  Threshold=0.5
  Tni : Gain  Gain=Tni
  TniRs_3 : Gain  Gain=Kpi
  Unit Delay : UnitDelay  SampleTime=-1
  _Tni : Gain  Gain=1/Tni
  dT_c : Constant  Value=T_ctrl  SampleTime=T_ctrl
  e_id : Sum  Inputs=+-
  id* : Constant  Value=0  SampleTime=T_ctrl
  int : Sum
  pi : Sum  Inputs=+++
  Data_bus : Outport
  u_ : Outport  Port=2
  d_id : Outport  Port=3
  wires:
  i/1 -> e_id/2, Bus Creator/3  "id_act[A]"
  Unit Delay/1 -> int/2
  Product/1 -> _Tni/1
  dT_c/1 -> Product/2
  pi/1 -> Switch_PI/1
  en_pi/1 -> Switch_PI/3, Switch_PI/2, Switch_I_Clr/2, Switch_I_Clr/3
  Switch_PI/1 -> u_/1, Bus Creator/1  "ud_pi[V]"
  _Tni/1 -> SwI/1
  en/1 -> SwI/3, SwI/2
  SwI/1 -> int/1
  int/1 -> Switch_I_Clr/1, pi/3
  Switch_I_Clr/1 -> Unit Delay/1
  del_ud/1 -> Tni/1
  Tni/1 -> Kf/1
  e_id/1 -> TniRs_3/1, d_id/1
  id_ref/1 -> Sel_Fw/2
  id*/1 -> Sel_Fw/3
  Sel_Fw/1 -> e_id/1, Bus Creator/2  "id_ref[A]"
  Kf/1 -> pi/1
  Sel_id_ref/1 -> Sel_Fw/1
  TniRs_3/1 -> Product/1, pi/2
  Bus Creator/1 -> Data_bus/1

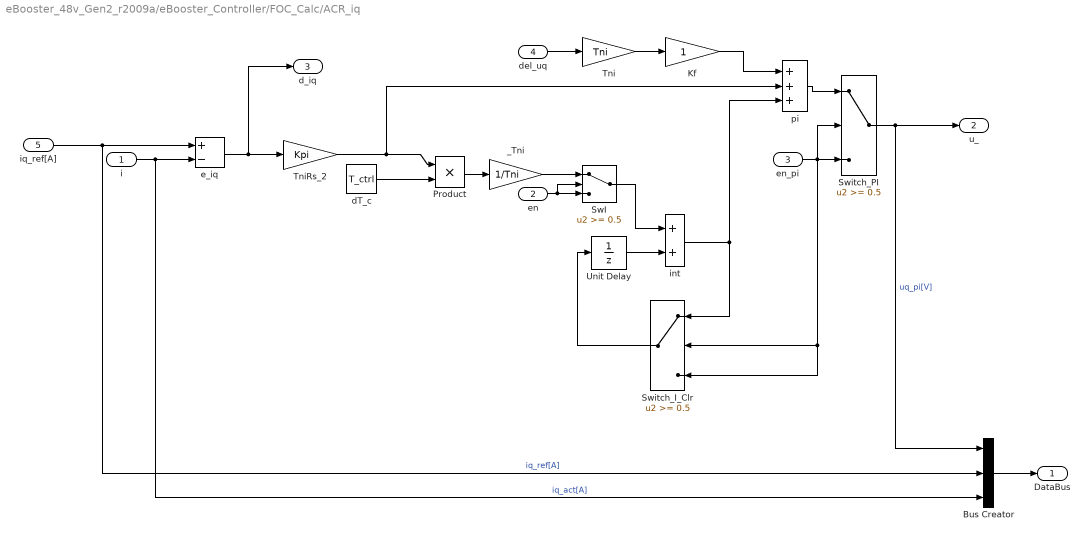
== system eBooster_48v_Gen2_r2009a/eBooster_Controller/FOC_Calc/ACR_iq ==
  i : Inport
  en : Inport  Port=2
  en_pi : Inport  Port=3
  del_uq : Inport  Port=4
  iq_ref[A] : Inport  Port=5
  Bus Creator : BusCreator  Inputs=3
  Kf : Gain
  Product : Product  RndMeth=Zero
  SwI : Switch  Threshold=0.5
  Switch_I_Clr : Switch  Threshold=0.5
  Switch_PI : Switch  Threshold=0.5
  Tni : Gain  Gain=Tni
  TniRs_2 : Gain  Gain=Kpi
  Unit Delay : UnitDelay  SampleTime=-1
  _Tni : Gain  Gain=1/Tni
  dT_c : Constant  Value=T_ctrl  SampleTime=T_ctrl
  e_iq : Sum  Inputs=+-
  int : Sum
  pi : Sum  Inputs=+++
  DataBus : Outport
  u_ : Outport  Port=2
  d_iq : Outport  Port=3
  wires:
  Switch_I_Clr/1 -> Unit Delay/1
  int/1 -> Switch_I_Clr/1, pi/3
  SwI/1 -> int/1
  en/1 -> SwI/2, SwI/3
  _Tni/1 -> SwI/1
  Switch_PI/1 -> u_/1, Bus Creator/1  "uq_pi[V]"
  en_pi/1 -> Switch_I_Clr/3, Switch_I_Clr/2, Switch_PI/2, Switch_PI/3
  pi/1 -> Switch_PI/1
  dT_c/1 -> Product/2
  Product/1 -> _Tni/1
  Unit Delay/1 -> int/2
  e_iq/1 -> d_iq/1, TniRs_2/1
  i/1 -> e_iq/2, Bus Creator/3  "iq_act[A]"
  Tni/1 -> Kf/1
  del_uq/1 -> Tni/1
  TniRs_2/1 -> Product/1, pi/2
  Kf/1 -> pi/1
  Bus Creator/1 -> DataBus/1
  iq_ref[A]/1 -> e_iq/1, Bus Creator/2  "iq_ref[A]"

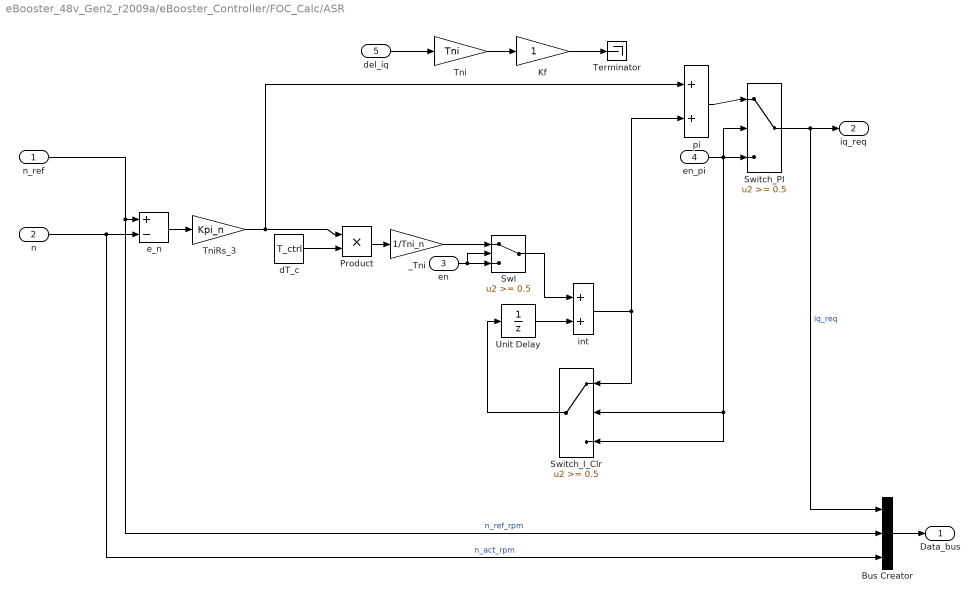
== system eBooster_48v_Gen2_r2009a/eBooster_Controller/FOC_Calc/ASR ==
  n_ref : Inport
  n : Inport  Port=2
  en : Inport  Port=3
  en_pi : Inport  Port=4
  del_iq : Inport  Port=5
  Bus Creator : BusCreator  Inputs=3
  Kf : Gain
  Product : Product  RndMeth=Zero
  SwI : Switch  Threshold=0.5
  Switch_I_Clr : Switch  Threshold=0.5
  Switch_PI : Switch  Threshold=0.5
  Terminator : Terminator
  Tni : Gain  Gain=Tni
  TniRs_3 : Gain  Gain=Kpi_n
  Unit Delay : UnitDelay  SampleTime=-1
  _Tni : Gain  Gain=1/Tni_n
  dT_c : Constant  Value=T_ctrl  SampleTime=T_ctrl
  e_n : Sum  Inputs=+-
  int : Sum
  pi : Sum
  Data_bus : Outport
  iq_req : Outport  Port=2
  wires:
  n/1 -> e_n/2, Bus Creator/3  "n_act_rpm"
  Unit Delay/1 -> int/2
  Product/1 -> _Tni/1
  dT_c/1 -> Product/2
  pi/1 -> Switch_PI/1
  en_pi/1 -> Switch_PI/3, Switch_PI/2, Switch_I_Clr/2, Switch_I_Clr/3
  Switch_PI/1 -> iq_req/1, Bus Creator/1  "iq_req"
  _Tni/1 -> SwI/1
  en/1 -> SwI/3, SwI/2
  SwI/1 -> int/1
  int/1 -> Switch_I_Clr/1, pi/2
  Switch_I_Clr/1 -> Unit Delay/1
  del_iq/1 -> Tni/1
  Tni/1 -> Kf/1
  e_n/1 -> TniRs_3/1
  n_ref/1 -> e_n/1, Bus Creator/2  "n_ref_rpm"
  TniRs_3/1 -> Product/1, pi/1
  Bus Creator/1 -> Data_bus/1
  Kf/1 -> Terminator/1

== system eBooster_48v_Gen2_r2009a/eBooster_Controller/FOC_Calc/FF ==
  we : Inport
  ctrl_id_bus : Inport  Port=2
  ctrl_iq_bus : Inport  Port=3
  Bus Creator : BusCreator  Inputs=3
  Bus Selector1 : BusSelector  OutputSignals=id_ref[A],id_act[A]
  Bus Selector2 : BusSelector  OutputSignals=iq_ref[A],iq_act[A]
  Ld : Gain  Gain=Ls
  Lq : Gain  Gain=Ls
  Sel_id : Switch  Threshold=0.5
  Sel_iq : Switch  Threshold=0.5
  Sw_ref_act : Constant
  min1 : Gain  Gain=-1
  psi_d : Bias  Bias=psi_p
  ud_ff : Product  RndMeth=Zero
  uq_ff2 : Product  RndMeth=Zero
  del_ud : Outport
  del_uq : Outport  Port=2
  DataBus : Outport  Port=3
  wires:
  ud_ff/1 -> min1/1
  we/1 -> ud_ff/1, uq_ff2/1, Bus Creator/1  "Speed_rad[s^-1]"
  Sel_iq/1 -> Lq/1, Bus Creator/3
  Lq/1 -> ud_ff/2
  min1/1 -> del_ud/1
  Sel_id/1 -> Ld/1, Bus Creator/2
  Ld/1 -> psi_d/1
  psi_d/1 -> uq_ff2/2
  uq_ff2/1 -> del_uq/1
  Bus Creator/1 -> DataBus/1
  ctrl_id_bus/1 -> Bus Selector1/1
  ctrl_iq_bus/1 -> Bus Selector2/1
  Bus Selector1/1 -> Sel_id/1  "<id_ref[A]>"
  Bus Selector1/2 -> Sel_id/3  "<id_act[A]>"
  Bus Selector2/1 -> Sel_iq/1  "<iq_ref[A]>"
  Bus Selector2/2 -> Sel_iq/3  "<iq_act[A]>"
  Sw_ref_act/1 -> Sel_id/2, Sel_iq/2

== system eBooster_48v_Gen2_r2009a/eBooster_Controller/FOC_Calc/FluxEstimator ==
  In1 : Inport
  Out1 : Outport
  wires:
  In1/1 -> Out1/1

== system eBooster_48v_Gen2_r2009a/eBooster_Controller/FOC_Calc/ParkTransformation ==
  cos/sin : Inport
  al/be : Inport  Port=2
  Bus Creator : BusCreator  Inputs='id[A]','iq[A]'
  Demux : Demux  Outputs=2
  Demux1 : Demux  Outputs=2
  al_cos : Product  RndMeth=Zero
  al_sin : Product  RndMeth=Zero
  be_cos : Product  RndMeth=Zero
  be_sin : Product  RndMeth=Zero
  id : Sum
  iq : Sum  Inputs=+-
  d/q : Outport
  wires:
  cos/sin/1 -> Demux/1
  al/be/1 -> Demux1/1
  Demux/1 -> al_cos/1, be_cos/2
  Demux1/1 -> al_cos/2, al_sin/1
  Demux/2 -> be_sin/1, al_sin/2
  Demux1/2 -> be_sin/2, be_cos/1
  al_cos/1 -> id/1
  be_sin/1 -> id/2
  be_cos/1 -> iq/1
  al_sin/1 -> iq/2
  Bus Creator/1 -> d/q/1
  id/1 -> Bus Creator/1  "id[A]"
  iq/1 -> Bus Creator/2  "iq[A]"

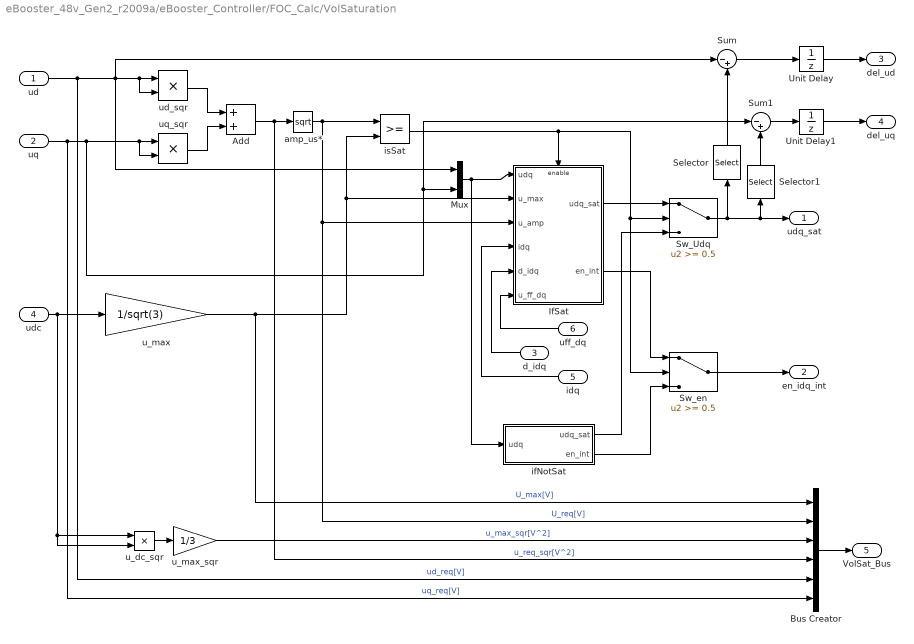
== system eBooster_48v_Gen2_r2009a/eBooster_Controller/FOC_Calc/VolSaturation ==
  ud : Inport
  uq : Inport  Port=2
  d_idq : Inport  Port=3
  udc : Inport  Port=4
  idq : Inport  Port=5
  uff_dq : Inport  Port=6
  Add : Sum
  Bus Creator : BusCreator  Inputs=6
  IfSat : Subsystem  TreatAsAtomicUnit=on
  Mux : Mux  Inputs=2
  Selector : Selector  InputPortWidth=2  IndexOptions=Index vector (dialog)  Indices=1  OutputSizes=1
  Selector1 : Selector  InputPortWidth=2  IndexOptions=Index vector (dialog)  Indices=2  OutputSizes=1
  Sum : Sum  Inputs=|-+
  Sum1 : Sum  Inputs=|-+
  Sw_Udq : Switch  Threshold=0.5
  Sw_en : Switch  Threshold=0.5
  Unit Delay : UnitDelay  SampleTime=-1
  Unit Delay1 : UnitDelay  SampleTime=-1
  amp_us* : Math  Operator=sqrt  SaturateOnIntegerOverflow=on
  ifNotSat : Subsystem  TreatAsAtomicUnit=on
  isSat : RelationalOperator  OutDataTypeStr=boolean
  u_dc_sqr : Product  RndMeth=Zero
  u_max : Gain  Gain=1/sqrt(3)
  u_max_sqr : Gain  Gain=1/3
  ud_sqr : Product  RndMeth=Zero
  uq_sqr : Product  RndMeth=Zero
  udq_sat : Outport
  en_idq_int : Outport  Port=2
  del_ud : Outport  Port=3
  del_uq : Outport  Port=4
  VolSat_Bus : Outport  Port=5
  wires:
  ud/1 -> ud_sqr/1, ud_sqr/2, Mux/1, Sum/1, Bus Creator/5  "ud_req[V]"
  uq/1 -> uq_sqr/1, uq_sqr/2, Mux/2, Sum1/1, Bus Creator/6  "uq_req[V]"
  ud_sqr/1 -> Add/1
  uq_sqr/1 -> Add/2
  udc/1 -> u_max/1, u_dc_sqr/1, u_dc_sqr/2
  Add/1 -> amp_us*/1, Bus Creator/4  "u_req_sqr[V^2]"
  amp_us*/1 -> isSat/1, IfSat/3(u_amp), Bus Creator/2  "U_req[V]"
  isSat/1 -> Sw_Udq/2, Sw_en/2, IfSat/Enable
  Mux/1 -> IfSat/1(udq), ifNotSat/1(udq)
  IfSat/1(udq_sat) -> Sw_Udq/1
  ifNotSat/1(udq_sat) -> Sw_Udq/3
  ifNotSat/2(en_int) -> Sw_en/3
  IfSat/2(en_int) -> Sw_en/1
  Sw_Udq/1 -> Selector/1, udq_sat/1, Selector1/1
  Sw_en/1 -> en_idq_int/1
  Sum/1 -> Unit Delay/1
  Sum1/1 -> Unit Delay1/1
  Selector/1 -> Sum/2
  Selector1/1 -> Sum1/2
  Unit Delay/1 -> del_ud/1
  Unit Delay1/1 -> del_uq/1
  idq/1 -> IfSat/4(idq)
  d_idq/1 -> IfSat/5(d_idq)
  uff_dq/1 -> IfSat/6(u_ff_dq)
  u_max/1 -> IfSat/2(u_max), isSat/2, Bus Creator/1  "U_max[V]"
  Bus Creator/1 -> VolSat_Bus/1
  u_dc_sqr/1 -> u_max_sqr/1
  u_max_sqr/1 -> Bus Creator/3  "u_max_sqr[V^2]"

== system eBooster_48v_Gen2_r2009a/eBooster_Controller/FOC_Calc/VoltageRegulator ==
  DataBusVolSat : Inport
  Bus Creator : BusCreator  Inputs=5
  Bus Selector1 : BusSelector  OutputSignals=u_max_sqr[V^2],u_req_sqr[V^2]
  I_max : Constant  Value=I_max
  PI : Subsystem
  SaturateIq : Subsystem  TreatAsAtomicUnit=on
  Saturation : Saturate  UpperLimit=0  LowerLimit=Id_ref_min
  Unit Delay : UnitDelay  SampleTime=-1
  en_avr : Constant  Value=en_avr
  isSaturated : RelationalOperator  Operator===  OutDataTypeStr=boolean
  id_ref : Outport
  iq_ref_lim : Outport  Port=2
  DataBus : Outport  Port=3
  wires:
  PI/1(i_d) -> isSaturated/1, Saturation/1
  Saturation/1 -> isSaturated/2, SaturateIq/2(Id_ref[A]), Bus Creator/1, id_ref/1  "id_ref[A]"
  isSaturated/1 -> Unit Delay/1
  Bus Selector1/1 -> PI/1(u_max), Bus Creator/2  "<u_max_sqr[V^2]>"
  Bus Selector1/2 -> PI/2(u_amp), Bus Creator/3  "<u_req_sqr[V^2]>"
  en_avr/1 -> PI/4(en_pi)
  Unit Delay/1 -> PI/3(en)
  I_max/1 -> SaturateIq/1(CAN_I_max[A])
  SaturateIq/1(Iq_sat[A]) -> iq_ref_lim/1, Bus Creator/4  "Iq_sat[A]"
  DataBusVolSat/1 -> Bus Selector1/1
  Bus Creator/1 -> DataBus/1

== system eBooster_48v_Gen2_r2009a/eBooster_Controller/MeasurementAndScaling/Iuvw_Meas1 ==
  note: -319A...319A
  note: Current scaling [A] --> digits
      | -319A...319A --> 0...1024
      | Note: Calibration not considered currently
  Iuvw[A] : Inport
  Bias : Bias  Bias=FOC_CURR_NULLIFICATION
  Data Type Conversion : DataTypeConversion  OutDataTypeStr=int16
  Gain : Gain  Gain=1/curr_adc_gain
  Saturation : Saturate  UpperLimit=319  LowerLimit=-319
  S16_Iuvw_ADC : Outport
  wires:
  Data Type Conversion/1 -> S16_Iuvw_ADC/1
  Bias/1 -> Data Type Conversion/1
  Gain/1 -> Bias/1
  Saturation/1 -> Gain/1
  Iuvw[A]/1 -> Saturation/1

== system eBooster_48v_Gen2_r2009a/eBooster_Controller/MeasurementAndScaling/_0_ADC_EVALUATION _1_CLARKE_TRANSFORMATION1 ==
  note: sint16
  note: W
  note: V
  note: U
  note: 1...6
  note: No FREEWHEELING and SYNC_CL States
  se_Sector : Inport
  i_uvw_adc : Inport  Port=2
  Demux : Demux  Outputs=3
  Merge : Merge  Inputs=3
  Merge1 : Merge  Inputs=3
  Mux1 : Mux  Inputs=2
  Mux2 : Mux  Inputs=2
  Mux3 : Mux  Inputs=2
  Switch Case : SwitchCase  CaseConditions={[1,6],[2,3],[4,5]}  ShowDefaultCase=off
  sector_1_6 : Subsystem  TreatAsAtomicUnit=on
  sector_2_3 : Subsystem  TreatAsAtomicUnit=on
  sector_4_5 : Subsystem  TreatAsAtomicUnit=on
  s_s16_I_alpha : Outport
  s_s16_I_beta : Outport  Port=2
  wires:
  Merge1/1 -> s_s16_I_beta/1
  sector_4_5/2(s_s16_I_beta) -> Merge1/3
  sector_2_3/2(s_s16_I_beta) -> Merge1/2
  sector_1_6/2(s_s16_I_beta) -> Merge1/1
  sector_4_5/1(s_s16_I_alpha) -> Merge/3
  sector_2_3/1(s_s16_I_alpha) -> Merge/2
  sector_1_6/1(s_s16_I_alpha) -> Merge/1
  Mux2/1 -> sector_4_5/1(In1)
  Demux/1 -> Mux2/1, Mux3/2
  Mux3/1 -> sector_2_3/1(In1)
  Demux/2 -> Mux2/2, Mux1/2
  Demux/3 -> Mux1/1, Mux3/1
  Mux1/1 -> sector_1_6/1(In1)
  Switch Case/3 -> sector_4_5/Action
  Switch Case/2 -> sector_2_3/Action
  Switch Case/1 -> sector_1_6/Action
  Merge/1 -> s_s16_I_alpha/1
  i_uvw_adc/1 -> Demux/1
  se_Sector/1 -> Switch Case/1

== system eBooster_48v_Gen2_r2009a/eBooster_Controller/FOC_Calc/VolSaturation/IfSat ==
  udq : Inport
  u_max : Inport  Port=2
  u_amp : Inport  Port=3
  idq : Inport  Port=4
  d_idq : Inport  Port=5
  u_ff_dq : Inport  Port=6
  Enable : EnablePort  PropagateVarSize=During execution
  Demux : Demux  Outputs=2
  Index Vector : MultiPortSwitch  zeroidx=off
  Mux : Mux  Inputs=2
  Mux1 : Mux  Inputs=2
  Mux2 : Mux  Inputs=2
  Sel_Sat : Constant  SampleTime=T_ctrl
  angle_method : Subsystem
  d_priority : Subsystem
  disInt : Constant  Value=[0 0]
  fac : Product  Inputs=*/
  ud_sat : Product  RndMeth=Zero
  uq_sat : Product  RndMeth=Zero
  udq_sat : Outport
  en_int : Outport  Port=2
  wires:
  disInt/1 -> en_int/1
  udq/1 -> Demux/1, d_priority/1(udq)
  u_max/1 -> fac/1, d_priority/2(u_max), angle_method/1(u_max)
  u_amp/1 -> fac/2
  Demux/1 -> ud_sat/1
  fac/1 -> ud_sat/2, uq_sat/2
  Demux/2 -> uq_sat/1
  ud_sat/1 -> Mux/1
  uq_sat/1 -> Mux/2
  d_priority/1(ud_sat) -> Mux1/1
  d_priority/2(uq_sat) -> Mux1/2
  Mux/1 -> Index Vector/2
  Mux1/1 -> Index Vector/3
  Index Vector/1 -> udq_sat/1
  Sel_Sat/1 -> Index Vector/1
  idq/1 -> angle_method/2(idq)
  angle_method/1(ud_sat) -> Mux2/1
  angle_method/2(uq_sat) -> Mux2/2
  Mux2/1 -> Index Vector/4
  d_idq/1 -> angle_method/3(d_idq)
  u_ff_dq/1 -> angle_method/4(u_ff_dq)

== system eBooster_48v_Gen2_r2009a/eBooster_Controller/FOC_Calc/VolSaturation/ifNotSat ==
  udq : Inport
  enInt : Constant  Value=[1 1]
  udq_sat : Outport
  en_int : Outport  Port=2
  wires:
  enInt/1 -> en_int/1
  udq/1 -> udq_sat/1

== system eBooster_48v_Gen2_r2009a/eBooster_Controller/FOC_Calc/VoltageRegulator/PI ==
  note: Manual Swich
      | Right Pos. Gain Scheduel
      | Left Pos. Constant Gain
  u_max : Inport
  u_amp : Inport  Port=2
  en : Inport  Port=3
  en_pi : Inport  Port=4
  Constant : Constant  Value=0
  Constant1 : Constant  Value=0
  Kpi_u : Gain  Gain=2^-4
  Kpi_u1 : Gain  Gain=2^-6
  SwI : Switch  Threshold=0.5
  Switch_I_Clr : Switch  Threshold=0.5
  Switch_PI : Switch  Threshold=0.5
  Unit Delay : UnitDelay  SampleTime=-1
  e_u_req : Sum  Inputs=+-
  int : Sum
  pi : Sum
  i_d : Outport
  wires:
  u_max/1 -> e_u_req/1
  Unit Delay/1 -> int/2
  pi/1 -> Switch_PI/1
  Switch_PI/1 -> i_d/1
  Kpi_u1/1 -> SwI/1
  en/1 -> SwI/3, SwI/2
  SwI/1 -> int/1
  int/1 -> pi/2, Switch_I_Clr/1
  Switch_I_Clr/1 -> Unit Delay/1
  e_u_req/1 -> Kpi_u1/1, Kpi_u/1
  u_amp/1 -> e_u_req/2
  en_pi/1 -> Switch_I_Clr/2, Switch_PI/2
  Constant/1 -> Switch_PI/3
  Constant1/1 -> Switch_I_Clr/3
  Kpi_u/1 -> pi/1

== system eBooster_48v_Gen2_r2009a/eBooster_Controller/FOC_Calc/VoltageRegulator/SaturateIq ==
  CAN_I_max[A] : Inport
  Id_ref[A] : Inport  Port=2
  AntiDivByZero : Saturate  UpperLimit=inf  LowerLimit=1
  Divide : Product  Inputs=*/
  Product : Product  RndMeth=Zero
  acos : Trigonometry  Operator=acos
  sin : Trigonometry
  Iq_sat[A] : Outport
  wires:
  Id_ref[A]/1 -> Divide/1
  CAN_I_max[A]/1 -> AntiDivByZero/1
  AntiDivByZero/1 -> Divide/2, Product/2
  Divide/1 -> acos/1
  acos/1 -> sin/1
  sin/1 -> Product/1
  Product/1 -> Iq_sat[A]/1
